simulink model "steering_pad_test"  (R2024b)
settings: Solver=VariableStepAuto  StartTime=0.0  StopTime=30  FixedStep=0.001  RelTol=1e-3
undefined symbols (not defined in the file): car
libraries: slpidlib x1, simulink x1, autolibshared x1
settings Model: Creator=Carlo  LastModifiedBy=HP

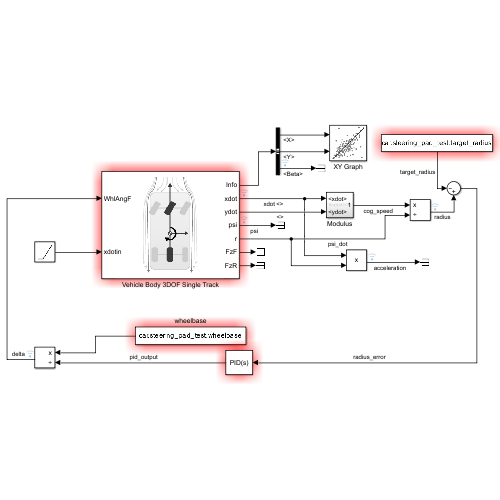
[thumbnail: Simulink's stored preview of the top-level diagram]
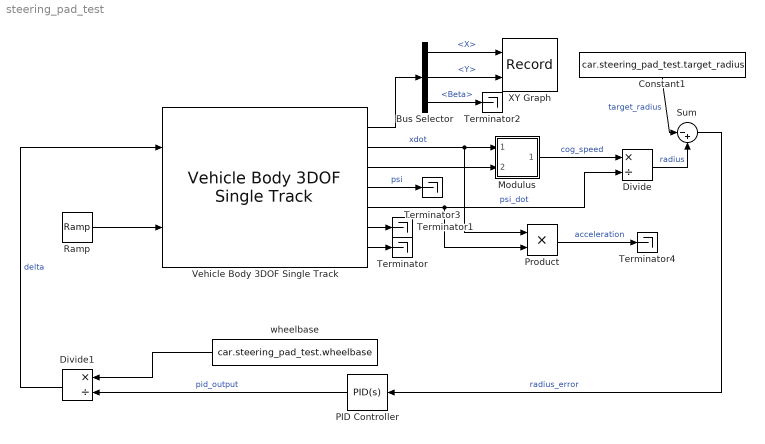
== system steering_pad_test ==
  Bus Selector : BusSelector  OutputSignals=InertFrm.Cg.Disp.X,InertFrm.Cg.Disp.Y,BdyFrm.Geom.Ang.Beta
  Constant1 : Constant  Value=car.steering_pad_test.target_radius
  Divide : Product  Inputs=*/
  Divide1 : Product  Inputs=*/
  Modulus : Subsystem
  PID Controller : slpidlib/PID Controller  Controller=PID  Form=Parallel  TimeDomain=Continuous-time  UseExternalTs=off  SampleTime=-1  IntegratorMethod=Forward Euler  FilterMethod=Forward Euler  ControllerParametersSource=internal  P=car.steering_pad_test.PID.P  I=car.steering_pad_test.PID.I  UseKiTs=off  D=car.steering_pad_test.PID.D  UseExternalDerivativeSource=off  N=car.steering_pad_test.PID.N  UseFilter=on  TunerSelectOption=Transfer Function Based (PID Tuner App)  InitialConditionSource=internal  InitialConditionForIntegrator=0  InitialConditionForFilter=0  DifferentiatorICPrevScaledInput=0  ExternalReset=none  TrackingMode=off  Kt=1  LimitOutput=off  SatLimitsSource=internal  UpperSaturationLimit=inf  LowerSaturationLimit=-inf  LinearizeAsGain=on  AntiWindupMode=none  Kb=1  LimitIntegrator=off  UpperIntegratorSaturationLimit=inf  LowerIntegratorSaturationLimit=-inf  POutMin=[]  POutMax=[]  IOutMin=[]  IOutMax=[]  DOutMin=[]  DOutMax=[]  NOutMin=[]  NOutMax=[]  SumOutMin=[]  SumOutMax=[]  SaturationOutMin=[]  SaturationOutMax=[]  PParamMin=[]  PParamMax=[]  IParamMin=[]  IParamMax=[]  DParamMin=[]  DParamMax=[]  NParamMin=[]  NParamMax=[]  KbParamMin=[]  KbParamMax=[]  KtParamMin=[]  KtParamMax=[]  KbOutMin=[]  KbOutMax=[]  KtOutMin=[]  KtOutMax=[]  IntegratorOutMin=[]  IntegratorOutMax=[]  FilterOutMin=[]  FilterOutMax=[]  SumI1OutMin=[]  SumI1OutMax=[]  SumI2OutMin=[]  SumI2OutMax=[]  SumI3OutMin=[]  SumI3OutMax=[]  SumI4OutMin=[]  SumI4OutMax=[]  SumDOutMin=[]  SumDOutMax=[]  DifferentiatorOutMin=[]  DifferentiatorOutMax=[]  FilterDiffOutCoefMin=[]  FilterDiffOutCoefMax=[]  ReciprocalOutMin=[]  ReciprocalOutMax=[]  SumDenOutMin=[]  SumDenOutMax=[]  SumNumOutMin=[]  SumNumOutMax=[]  DivideOutMin=[]  DivideOutMax=[]  UdiffTsProdOutMin=[]  UdiffTsProdOutMax=[]  NTsProdOutMin=[]  NTsProdOutMax=[]  UintegralTsProdOutMin=[]  UintegralTsProdOutMax=[]  UngainTsProdOutMin=[]  UngainTsProdOutMax=[]  ClampingZeroOutDataTypeStr=Inherit: Inherit via back propagation  ClampingZeroOutMin=[]  ClampingZeroOutMax=[]  FilterDenConstantOutDataTypeStr=Inherit: Inherit via back propagation  FilterDenConstantOutMin=[]  FilterDenConstantOutMax=[]  PCopyOutDataTypeStr=Inherit: Inherit via back propagation  PCopyOutMin=[]  PCopyOutMax=[]  NCopyOutDataTypeStr=Inherit: Inherit via back propagation  NCopyOutMin=[]  NCopyOutMax=[]  IntegratorContinuousStateAttributes=''  IntegratorStateMustResolveToSignalObject=off  IntegratorRTWStateStorageClass=Auto  FilterContinuousStateAttributes=''  FilterStateMustResolveToSignalObject=off  FilterRTWStateStorageClass=Auto  ParallelPVariant=InternalParameters  IdealPVariant=Disabled  IVariant=InternalParameters  DVariant=InternalParameters  IntegratorVariant=Continuous  SatVariant=Disabled  AWVariant=Passthrough  PCopyVariant=Disabled  TRVariant=Disabled  FdbkBlocksVariant=Forward  IdealPFdbkVariant=Disabled  SatFdbkVariant=Disabled  DerivativeFilterVariant=ContFilter  NVariant=InternalParameters  NCopyVariant=Disabled  FilterICVariant=InternalICsFilter  IntegratorICVariant=InternalICs  ExternalResetVariant=Disabled  TRSumVariant=Passthrough  SumFdbkVariant=Disabled  SumVariant=Sum_PID  TsampFilterVariant=InternalTs  TsampNgainVariant=Passthrough  TsampIntegralVariant=Disabled_SignalSpec  ExternalSaturationOutDataTypeStr=Inherit: Same as second input  DerivativeSourceVariant=ErrorSignal  PreIntVariant=InternalPreInt
  Product : Product
  Ramp : simulink/Sources/Ramp  slope=0.6  start=0  InitialOutput=2
  Sum : Sum  Inputs=|-+
  Terminator{,1..4} (5 alike) : Terminator
  Vehicle Body 3DOF Single Track : autolibshared/Vehicle Body 3DOF Single Track  trackMode=Single (bicycle)  inputMode=External longitudinal velocity  frontSteerMode=on  rearSteerMode=off  windMode=off  muMode=off  extFMode=off  extMMode=off  htchFMode=off  htchMMode=off  extXo=off  extpsio=off  extxdoto=off  extro=off  extYo=off  extTamb=off  extydoto=off  aMode=2  NF=car.lateralbody.NF  NR=car.lateralbody.NR  m=car.lateralbody.m  a=car.lateralbody.a  b=car.lateralbody.b  h=car.lateralbody.h  dh=1  hh=0.2  X_o=car.lateralbody.X_o  xdot_o=5  CalphaMode=off  sigmaMode=on  d=0  hl=0  w=[1.4,1.4]  Cy_f=car.lateralbody.Cy_f  Cy_r=car.lateralbody.Cy_r  sigma_f=car.lateralbody.sigma_f  sigma_r=car.lateralbody.sigma_r  alpha_f_brk=[-.1 .1]  Cy_f_data=[-9e3 9e3]  alpha_r_brk=[-.1 .1]  Cy_r_data=[-9e3 9e3]  Y_o=car.lateralbody.Y_o  ydot_o=car.lateralbody.ydot_o  Izz=car.lateralbody.Izz  psi_o=car.lateralbody.psi_o  r_o=car.lateralbody.r_o  Af=car.lateralbody.Af  Cd=car.lateralbody.Cd  Cl=car.lateralbody.Cl  Cpm=car.lateralbody.Cpm  beta_w=car.lateralbody.beta_w  Cs=car.lateralbody.Cs  Cym=car.lateralbody.Cym  Pabs=car.lateralbody.Pabs  Tair=car.lateralbody.Tair  g=car.lateralbody.g  mu=car.lateralbody.mu  xdot_tol=car.lateralbody.xdot_tol  Fznom=car.lateralbody.Fznom  Fxtire_sat=7e4  Fytire_sat=7e4  longOff=car.lateralbody.longOff  latOff=car.lateralbody.latOff  vertOff=car.lateralbody.vertOff  wrapAng=off
      settings: LibrarySourceBlock=vehdynlibeom/Vehicle Body 3DOF Dual Track
  XY Graph : Record  FileSettingsInternal="{\"entries\":[{\"content\":{\"excelSettings\":{\"content\":{},\"type\":\"Streamout.ExcelSettings\"}},\"type\":\"Streamout.FileSettingStorage\",\"uuid\":\"\"}],\"packageUris\":[\"http:\\/\\/schema.mathworks.com\\/mf0\\/streamout_blocks\\/R2020a\"],\"version\":\"1.0\"}"  Layout=[1 1]  SignalsInternal="{\"entries\":[{\"content\":{\"signals\":[{\"content\":{\"blockPath\":[],\"dimensions\":[1],\"domain\":\"\",\"lineColor\":\"#a2142f\",\"plots\":[ 1 ],\"port\":1,\"signalID\":1,\"signalName\":\"<X>\"},\"type\":\"RecordBlkView.Signal\",\"uuid\":\"\"},{\"content\":{\"blockPath\":[],\"dimensions\":[1],\"domain\":\"\",\"lineColor\":\"#fe330a\",\"plots\":[ 1 ],\"port\":2,\"signalID\":2,\"signalName\":\"<Y>\"},\"type\":\"RecordBlkView.Signal\",\"uuid\":\"\"}]},\"type\":\"RecordBlkView.InputSignals\",\"uuid\":\"\"}],\"packageUris\":[\"http:\\/\\/schema.mathworks.com\\/mf0\\/streamout_blocks\\/R2020a\"],\"version\":\"1.0\"}"  VisualizationBindings="{\"xyplotplugin\":{\"info\":[{\"series\":[{\"bindingParametersList\":[{\"parameter\":\"X-Axis\",\"signalID\":1,\"signalName\":\"<X>\"},{\"parameter\":\"Y-Axis\",\"signalID\":2,\"signalName\":\"<Y>\"}],\"seriesID\":0},{\"bindingParametersList\":[{\"parameter\":\"X-Axis\",\"signalID\":1,\"signalName\":\"<X>\"}],\"seriesID\":1}],\"subplotID\":1}]}}"  CompatibilityTag=XY
  wheelbase : Constant  Value=car.steering_pad_test.wheelbase
  wires:
  Vehicle Body 3DOF Single Track/7 -> Terminator/1
  Vehicle Body 3DOF Single Track/6 -> Terminator1/1
  Vehicle Body 3DOF Single Track/5 -> Product/2, Divide/2  "psi_dot"
  Vehicle Body 3DOF Single Track/4 -> Terminator3/1  "psi"
  Vehicle Body 3DOF Single Track/1 -> Bus Selector/1
  Bus Selector/1 -> XY Graph/1  "<X>"
  Bus Selector/2 -> XY Graph/2  "<Y>"
  Vehicle Body 3DOF Single Track/2 -> Product/1, Modulus/1(<xdot>)  "xdot"
  Vehicle Body 3DOF Single Track/3 -> Modulus/2(<ydot>)
  Modulus/1(Out1) -> Divide/1  "cog_speed"
  Divide/1 -> Sum/2  "radius"
  Sum/1 -> PID Controller/1  "radius_error"
  wheelbase/1 -> Divide1/1
  Divide1/1 -> Vehicle Body 3DOF Single Track/1  "delta"
  PID Controller/1 -> Divide1/2  "pid_output"
  Bus Selector/3 -> Terminator2/1  "<Beta>"
  Product/1 -> Terminator4/1  "acceleration"
  Ramp/1 -> Vehicle Body 3DOF Single Track/2
  Constant1/1 -> Sum/1  "target_radius"

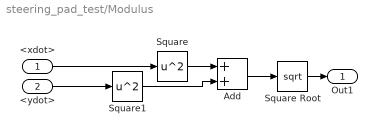
== system steering_pad_test/Modulus ==
  <xdot> : Inport
  <ydot> : Inport  Port=2
  Add : Sum
  Square : Math  Operator=square
  Square Root : Sqrt
  Square1 : Math  Operator=square
  Out1 : Outport
  wires:
  Add/1 -> Square Root/1
  Square/1 -> Add/1
  Square1/1 -> Add/2
  Square Root/1 -> Out1/1
  <ydot>/1 -> Square1/1
  <xdot>/1 -> Square/1
